simulink model "iControlLogic"  (R2017b)
settings: Solver=VariableStepAuto  StartTime=0.0  StopTime=10.0  RelTol=1e-3
settings Model: Creator=ohm9xd  LastModifiedBy=ohm9xd

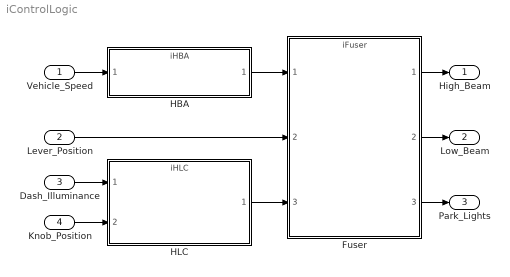
== system iControlLogic ==
  Vehicle_Speed : Inport
  Lever_Position : Inport  Port=2
  Dash_Illuminance : Inport  Port=3
  Knob_Position : Inport  Port=4
  Fuser : ModelReference  ModelNameDialog=iFuser.slx  SimulationMode=Normal  ModelReferenceVersion=1.1
  HBA : ModelReference  ModelNameDialog=iHBA.slx  SimulationMode=Normal  ModelReferenceVersion=1.1
  HLC : ModelReference  ModelNameDialog=iHLC.slx  SimulationMode=Normal  ModelReferenceVersion=1.1
  High_Beam : Outport
  Low_Beam : Outport  Port=2
  Park_Lights : Outport  Port=3
  wires:
  Fuser/2 -> Low_Beam/1
  Fuser/3 -> Park_Lights/1
  Fuser/1 -> High_Beam/1
  HBA/1 -> Fuser/1
  Vehicle_Speed/1 -> HBA/1
  Lever_Position/1 -> Fuser/2
  HLC/1 -> Fuser/3
  Dash_Illuminance/1 -> HLC/1
  Knob_Position/1 -> HLC/2
